simulink model "simu2"  (R2024a)
settings: Solver=VariableStepAuto  StartTime=0.0  StopTime=10.0  RelTol=1e-3
undefined symbols (not defined in the file or in its folder): A, B, C, D, r
settings Model: Creator=simon  LastModifiedBy=simon

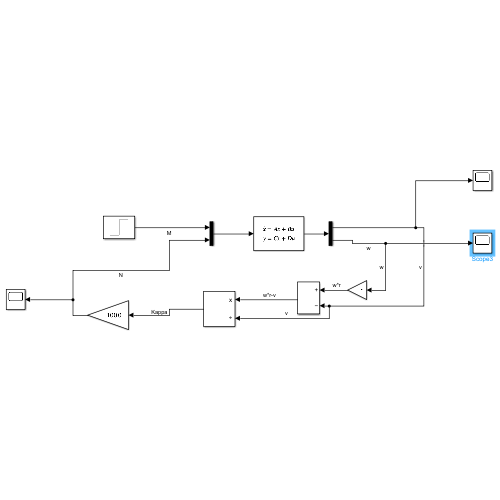
[thumbnail: Simulink's stored preview of the top-level diagram]
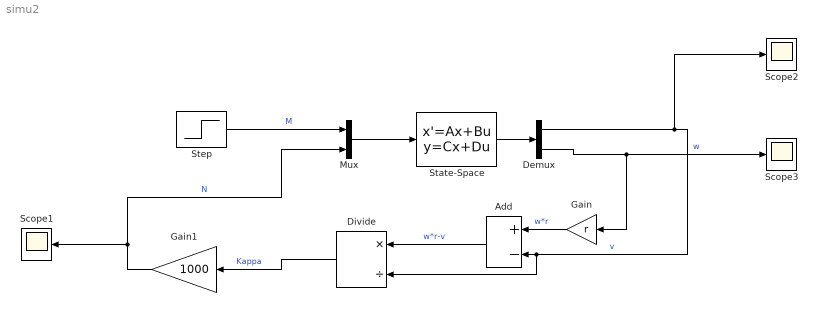
== system simu2 ==
  Add : Sum  Inputs=+-
  Demux : Demux  Outputs=2
  Divide : Product  Inputs=*/
  Gain : Gain  Gain=r
  Gain1 : Gain  Gain=1000
  Mux : Mux  Inputs=2
  Scope1 : Scope
  Scope2 : Scope
  Scope3 : Scope
  State-Space : StateSpace  A=A  B=B  C=C  D=D  InitialCondition=[0.1 0.1/r]
  Step : Step  After=1000  SampleTime=0
  wires:
  Mux/1 -> State-Space/1
  State-Space/1 -> Demux/1
  Step/1 -> Mux/1  "M"
  Demux/1 -> Scope2/1, Divide/2, Add/2  "v"
  Demux/2 -> Scope3/1, Gain/1  "w"
  Gain/1 -> Add/1  "w*r"
  Add/1 -> Divide/1  "w*r-v"
  Divide/1 -> Gain1/1  "Kappa"
  Gain1/1 -> Scope1/1, Mux/2  "N"
